simulink model "COMPLETETEST_InDividualLegControl"  (R2023a)
settings: Solver=VariableStepAuto  StartTime=0.0  StopTime=80.0  RelTol=1e-3
undefined symbols (not defined in the file or in its folder): X, Y, Z
libraries: sm_lib x95, simulink_extras x24, nesl_utility x10
(part 3 of 3)

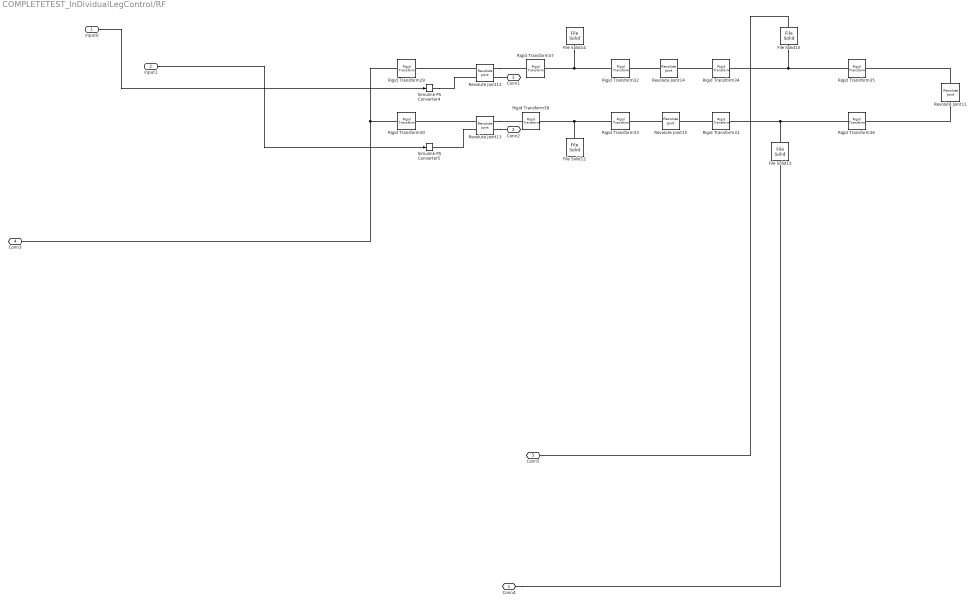
== system COMPLETETEST_InDividualLegControl/RF ==
  input0 : Inport
  input1 : Inport  Port=2
  File Solid12 : sm_lib/Body Elements/File Solid  ExtGeomFileName=F:\THE_LIBRARY\CODE_BASE\ROBOSERVO\Odrive\TINDALOS_THEDOG\SIM_MATLAB\ABSTARCT\LINK1.STL  UnitType=Custom  ExtGeomFileUnits=mm  StepReaderType=HEX  ExportConvexHullGeometry=off  InertiaType=CalculateFromGeometry  Mass=1  MassUnits=kg  CenterOfMass=[0 0 0]  CenterOfMassUnits=m  MomentsOfInertia=[1 1 1]  MomentsOfInertiaUnits=kg*m^2  ProductsOfInertia=[0 0 0]  ProductsOfInertiaUnits=kg*m^2  BasedOnType=Density  Density=1000  DensityUnits=kg/m^3  DoExposeReferenceFrame=on  SerializedFrames=<Frames/>  GraphicType=FromGeometry  MarkerShape=Sphere  MarkerSize=10  GraphicVisPropType=SimpleVisualProperties  GraphicDiffuseColor=[1.0 0.2 0.2]  GraphicSpecularColor=[0.5 0.5 0.5 1.0]  GraphicAmbientColor=[0.15 0.15 0.15 1.0]  GraphicEmissiveColor=[0.0 0.0 0.0 1.0]  GraphicShininess=75  GraphicOpacity=1.0
  File Solid13 : sm_lib/Body Elements/File Solid  ExtGeomFileName=F:\THE_LIBRARY\CODE_BASE\ROBOSERVO\Odrive\TINDALOS_THEDOG\SIM_MATLAB\ABSTARCT\LINK2.STL  UnitType=Custom  ExtGeomFileUnits=mm  StepReaderType=HEX  ExportConvexHullGeometry=on  InertiaType=CalculateFromGeometry  Mass=1  MassUnits=kg  CenterOfMass=[0 0 0]  CenterOfMassUnits=m  MomentsOfInertia=[1 1 1]  MomentsOfInertiaUnits=kg*m^2  ProductsOfInertia=[0 0 0]  ProductsOfInertiaUnits=kg*m^2  BasedOnType=Density  Density=1000  DensityUnits=kg/m^3  DoExposeReferenceFrame=on  SerializedFrames=<Frames/>  GraphicType=FromGeometry  MarkerShape=Sphere  MarkerSize=10  GraphicVisPropType=SimpleVisualProperties  GraphicDiffuseColor=[1.0 0.6 0.0]  GraphicSpecularColor=[0.5 0.5 0.5 1.0]  GraphicAmbientColor=[0.15 0.15 0.15 1.0]  GraphicEmissiveColor=[0.0 0.0 0.0 1.0]  GraphicShininess=75  GraphicOpacity=1.0
  File Solid14 : sm_lib/Body Elements/File Solid  ExtGeomFileName=F:\THE_LIBRARY\CODE_BASE\ROBOSERVO\Odrive\TINDALOS_THEDOG\SIM_MATLAB\ABSTARCT\LINK1.STL  UnitType=Custom  ExtGeomFileUnits=mm  StepReaderType=HEX  ExportConvexHullGeometry=off  InertiaType=CalculateFromGeometry  Mass=1  MassUnits=kg  CenterOfMass=[0 0 0]  CenterOfMassUnits=m  MomentsOfInertia=[1 1 1]  MomentsOfInertiaUnits=kg*m^2  ProductsOfInertia=[0 0 0]  ProductsOfInertiaUnits=kg*m^2  BasedOnType=Density  Density=1000  DensityUnits=kg/m^3  DoExposeReferenceFrame=on  SerializedFrames=<Frames/>  GraphicType=FromGeometry  MarkerShape=Sphere  MarkerSize=10  GraphicVisPropType=SimpleVisualProperties  GraphicDiffuseColor=[1.0 0.2 0.2]  GraphicSpecularColor=[0.5 0.5 0.5 1.0]  GraphicAmbientColor=[0.15 0.15 0.15 1.0]  GraphicEmissiveColor=[0.0 0.0 0.0 1.0]  GraphicShininess=75  GraphicOpacity=1.0
  File Solid15 : sm_lib/Body Elements/File Solid  ExtGeomFileName=F:\THE_LIBRARY\CODE_BASE\ROBOSERVO\Odrive\TINDALOS_THEDOG\SIM_MATLAB\ABSTARCT\LINK2.STL  UnitType=Custom  ExtGeomFileUnits=mm  StepReaderType=HEX  ExportConvexHullGeometry=on  InertiaType=CalculateFromGeometry  Mass=1  MassUnits=kg  CenterOfMass=[0 0 0]  CenterOfMassUnits=m  MomentsOfInertia=[1 1 1]  MomentsOfInertiaUnits=kg*m^2  ProductsOfInertia=[0 0 0]  ProductsOfInertiaUnits=kg*m^2  BasedOnType=Density  Density=1000  DensityUnits=kg/m^3  DoExposeReferenceFrame=on  SerializedFrames=<Frames/>  GraphicType=FromGeometry  MarkerShape=Sphere  MarkerSize=10  GraphicVisPropType=SimpleVisualProperties  GraphicDiffuseColor=[1.0 0.6 0.0]  GraphicSpecularColor=[0.5 0.5 0.5 1.0]  GraphicAmbientColor=[0.15 0.15 0.15 1.0]  GraphicEmissiveColor=[0.0 0.0 0.0 1.0]  GraphicShininess=75  GraphicOpacity=1.0
  Revolute Joint11 : sm_lib/Joints/Revolute Joint  JointMode=Normal  SenseConstraintForce=off  SenseConstraintForceX=off  SenseConstraintForceY=off  SenseConstraintForceZ=off  SenseConstraintTorque=off  SenseConstraintTorqueX=off  SenseConstraintTorqueY=off  SenseConstraintTorqueZ=off  SenseTotalForce=off  SenseTotalForceX=off  SenseTotalForceY=off  SenseTotalForceZ=off  SenseTotalTorque=off  SenseTotalTorqueX=off  SenseTotalTorqueY=off  SenseTotalTorqueZ=off  CompositeWrenchDir=FollowerOnBase  CompositeWrenchFrame=BaseFrame  EquilibriumPosition=0  EquilibriumPositionUnits=deg  SpringStiffness=0  SpringStiffnessUnits=N*m/deg  DampingCoefficient=0  DampingCoefficientUnits=N*m/(deg/s)  TorqueActuationMode=NoTorque  MotionActuationMode=ComputedMotion  SensePosition=off  SenseVelocity=off  SenseAcceleration=off  SenseTorqueForce=off  SenseLowerLimitTorqueForce=off  SenseUpperLimitTorqueForce=off  LowerLimitSpecify=off  LowerLimitBound=-90  LowerLimitBoundUnits=deg  LowerLimitStiffness=1e4  LowerLimitStiffnessUnits=N*m/deg  LowerLimitDamping=10  LowerLimitDampingUnits=N*m/(deg/s)  LowerLimitTransitionRegionWidth=0.1  LowerLimitTransitionRegionWidthUnits=deg  UpperLimitSpecify=off  UpperLimitBound=90  UpperLimitBoundUnits=deg  UpperLimitStiffness=1e4  UpperLimitStiffnessUnits=N*m/deg  UpperLimitDamping=10  UpperLimitDampingUnits=N*m/(deg/s)  UpperLimitTransitionRegionWidth=0.1  UpperLimitTransitionRegionWidthUnits=deg  PositionTargetSpecify=off  PositionTargetPriority=High  PositionTargetValue=0  PositionTargetValueUnits=deg  VelocityTargetSpecify=off  VelocityTargetPriority=High  VelocityTargetValue=0  VelocityTargetValueUnits=deg/s
  Revolute Joint12 : sm_lib/Joints/Revolute Joint  JointMode=Normal  SenseConstraintForce=off  SenseConstraintForceX=off  SenseConstraintForceY=off  SenseConstraintForceZ=off  SenseConstraintTorque=off  SenseConstraintTorqueX=off  SenseConstraintTorqueY=off  SenseConstraintTorqueZ=off  SenseTotalForce=off  SenseTotalForceX=off  SenseTotalForceY=off  SenseTotalForceZ=off  SenseTotalTorque=off  SenseTotalTorqueX=off  SenseTotalTorqueY=off  SenseTotalTorqueZ=off  CompositeWrenchDir=FollowerOnBase  CompositeWrenchFrame=BaseFrame  EquilibriumPosition=0  EquilibriumPositionUnits=deg  SpringStiffness=0  SpringStiffnessUnits=N*m/deg  DampingCoefficient=1e-4  DampingCoefficientUnits=N*m/(deg/s)  TorqueActuationMode=ComputedTorque  MotionActuationMode=InputMotion  SensePosition=on  SenseVelocity=off  SenseAcceleration=off  SenseTorqueForce=off  SenseLowerLimitTorqueForce=off  SenseUpperLimitTorqueForce=off  LowerLimitSpecify=off  LowerLimitBound=-90  LowerLimitBoundUnits=deg  LowerLimitStiffness=1e4  LowerLimitStiffnessUnits=N*m/deg  LowerLimitDamping=10  LowerLimitDampingUnits=N*m/(deg/s)  LowerLimitTransitionRegionWidth=0.1  LowerLimitTransitionRegionWidthUnits=deg  UpperLimitSpecify=off  UpperLimitBound=90  UpperLimitBoundUnits=deg  UpperLimitStiffness=1e4  UpperLimitStiffnessUnits=N*m/deg  UpperLimitDamping=10  UpperLimitDampingUnits=N*m/(deg/s)  UpperLimitTransitionRegionWidth=0.1  UpperLimitTransitionRegionWidthUnits=deg  PositionTargetSpecify=off  PositionTargetPriority=High  PositionTargetValue=120  PositionTargetValueUnits=deg  VelocityTargetSpecify=off  VelocityTargetPriority=High  VelocityTargetValue=0  VelocityTargetValueUnits=deg/s
  Revolute Joint13 : sm_lib/Joints/Revolute Joint  JointMode=Normal  SenseConstraintForce=off  SenseConstraintForceX=off  SenseConstraintForceY=off  SenseConstraintForceZ=off  SenseConstraintTorque=off  SenseConstraintTorqueX=off  SenseConstraintTorqueY=off  SenseConstraintTorqueZ=off  SenseTotalForce=off  SenseTotalForceX=off  SenseTotalForceY=off  SenseTotalForceZ=off  SenseTotalTorque=off  SenseTotalTorqueX=off  SenseTotalTorqueY=off  SenseTotalTorqueZ=off  CompositeWrenchDir=FollowerOnBase  CompositeWrenchFrame=BaseFrame  EquilibriumPosition=0  EquilibriumPositionUnits=deg  SpringStiffness=0  SpringStiffnessUnits=N*m/deg  DampingCoefficient=1e-4  DampingCoefficientUnits=N*m/(deg/s)  TorqueActuationMode=ComputedTorque  MotionActuationMode=InputMotion  SensePosition=on  SenseVelocity=off  SenseAcceleration=off  SenseTorqueForce=off  SenseLowerLimitTorqueForce=off  SenseUpperLimitTorqueForce=off  LowerLimitSpecify=off  LowerLimitBound=-90  LowerLimitBoundUnits=deg  LowerLimitStiffness=1e4  LowerLimitStiffnessUnits=N*m/deg  LowerLimitDamping=10  LowerLimitDampingUnits=N*m/(deg/s)  LowerLimitTransitionRegionWidth=0.1  LowerLimitTransitionRegionWidthUnits=deg  UpperLimitSpecify=off  UpperLimitBound=90  UpperLimitBoundUnits=deg  UpperLimitStiffness=1e4  UpperLimitStiffnessUnits=N*m/deg  UpperLimitDamping=10  UpperLimitDampingUnits=N*m/(deg/s)  UpperLimitTransitionRegionWidth=0.1  UpperLimitTransitionRegionWidthUnits=deg  PositionTargetSpecify=off  PositionTargetPriority=High  PositionTargetValue=-60  PositionTargetValueUnits=deg  VelocityTargetSpecify=off  VelocityTargetPriority=High  VelocityTargetValue=0  VelocityTargetValueUnits=deg/s
  Revolute Joint14 : sm_lib/Joints/Revolute Joint  JointMode=Normal  SenseConstraintForce=off  SenseConstraintForceX=off  SenseConstraintForceY=off  SenseConstraintForceZ=off  SenseConstraintTorque=off  SenseConstraintTorqueX=off  SenseConstraintTorqueY=off  SenseConstraintTorqueZ=off  SenseTotalForce=off  SenseTotalForceX=off  SenseTotalForceY=off  SenseTotalForceZ=off  SenseTotalTorque=off  SenseTotalTorqueX=off  SenseTotalTorqueY=off  SenseTotalTorqueZ=off  CompositeWrenchDir=FollowerOnBase  CompositeWrenchFrame=BaseFrame  EquilibriumPosition=0  EquilibriumPositionUnits=deg  SpringStiffness=0  SpringStiffnessUnits=N*m/deg  DampingCoefficient=0  DampingCoefficientUnits=N*m/(deg/s)  TorqueActuationMode=NoTorque  MotionActuationMode=ComputedMotion  SensePosition=off  SenseVelocity=off  SenseAcceleration=off  SenseTorqueForce=off  SenseLowerLimitTorqueForce=off  SenseUpperLimitTorqueForce=off  LowerLimitSpecify=off  LowerLimitBound=-90  LowerLimitBoundUnits=deg  LowerLimitStiffness=1e4  LowerLimitStiffnessUnits=N*m/deg  LowerLimitDamping=10  LowerLimitDampingUnits=N*m/(deg/s)  LowerLimitTransitionRegionWidth=0.1  LowerLimitTransitionRegionWidthUnits=deg  UpperLimitSpecify=off  UpperLimitBound=90  UpperLimitBoundUnits=deg  UpperLimitStiffness=1e4  UpperLimitStiffnessUnits=N*m/deg  UpperLimitDamping=10  UpperLimitDampingUnits=N*m/(deg/s)  UpperLimitTransitionRegionWidth=0.1  UpperLimitTransitionRegionWidthUnits=deg  PositionTargetSpecify=off  PositionTargetPriority=Low  PositionTargetValue=-135  PositionTargetValueUnits=deg  VelocityTargetSpecify=off  VelocityTargetPriority=High  VelocityTargetValue=90  VelocityTargetValueUnits=deg/s
  Revolute Joint15 : sm_lib/Joints/Revolute Joint  JointMode=Normal  SenseConstraintForce=off  SenseConstraintForceX=off  SenseConstraintForceY=off  SenseConstraintForceZ=off  SenseConstraintTorque=off  SenseConstraintTorqueX=off  SenseConstraintTorqueY=off  SenseConstraintTorqueZ=off  SenseTotalForce=off  SenseTotalForceX=off  SenseTotalForceY=off  SenseTotalForceZ=off  SenseTotalTorque=off  SenseTotalTorqueX=off  SenseTotalTorqueY=off  SenseTotalTorqueZ=off  CompositeWrenchDir=FollowerOnBase  CompositeWrenchFrame=BaseFrame  EquilibriumPosition=0  EquilibriumPositionUnits=deg  SpringStiffness=0  SpringStiffnessUnits=N*m/deg  DampingCoefficient=0  DampingCoefficientUnits=N*m/(deg/s)  TorqueActuationMode=NoTorque  MotionActuationMode=ComputedMotion  SensePosition=off  SenseVelocity=off  SenseAcceleration=off  SenseTorqueForce=off  SenseLowerLimitTorqueForce=off  SenseUpperLimitTorqueForce=off  LowerLimitSpecify=off  LowerLimitBound=-90  LowerLimitBoundUnits=deg  LowerLimitStiffness=1e4  LowerLimitStiffnessUnits=N*m/deg  LowerLimitDamping=10  LowerLimitDampingUnits=N*m/(deg/s)  LowerLimitTransitionRegionWidth=0.1  LowerLimitTransitionRegionWidthUnits=deg  UpperLimitSpecify=off  UpperLimitBound=90  UpperLimitBoundUnits=deg  UpperLimitStiffness=1e4  UpperLimitStiffnessUnits=N*m/deg  UpperLimitDamping=10  UpperLimitDampingUnits=N*m/(deg/s)  UpperLimitTransitionRegionWidth=0.1  UpperLimitTransitionRegionWidthUnits=deg  PositionTargetSpecify=off  PositionTargetPriority=Low  PositionTargetValue=-135  PositionTargetValueUnits=deg  VelocityTargetSpecify=off  VelocityTargetPriority=High  VelocityTargetValue=90  VelocityTargetValueUnits=deg/s
  Rigid Transform29 : sm_lib/Frames and Transforms/Rigid Transform  TranslationMethod=StandardAxis  TranslationStandardOffset=6  TranslationStandardOffsetUnits=mm  TranslationStandardAxis=+Z  TranslationCartesianOffset=[0 0 0]  TranslationCartesianOffsetUnits=m  TranslationROffset=0  TranslationROffsetUnits=m  TranslationZOffset=0  TranslationZOffsetUnits=m  TranslationThetaOffset=0  TranslationThetaOffsetUnits=deg  RotationMethod=None  RotationAngleUnits=deg  RotationStandardAxis=+X  RotationAngle=90  RotationArbitraryAxis=[0 0 1]  FollAlignAxisA=+X  BaseAlignAxisA=+Y  FollAlignAxisB=+Y  BaseAlignAxisB=+Z  RotationSequenceAxes=FollowerAxes  RotationSequence=XYX  RotationSequenceAngles=[0 0 0]  RotationSequenceAnglesUnits=deg  RotationMatrix=[1 0 0; 0 1 0; 0 0 1]  Quaternion=[1 0 0 0]
  Rigid Transform30 : sm_lib/Frames and Transforms/Rigid Transform  TranslationMethod=StandardAxis  TranslationStandardOffset=6  TranslationStandardOffsetUnits=mm  TranslationStandardAxis=-Z  TranslationCartesianOffset=[0 0 0]  TranslationCartesianOffsetUnits=m  TranslationROffset=0  TranslationROffsetUnits=m  TranslationZOffset=0  TranslationZOffsetUnits=m  TranslationThetaOffset=0  TranslationThetaOffsetUnits=deg  RotationMethod=None  RotationAngleUnits=deg  RotationStandardAxis=+X  RotationAngle=90  RotationArbitraryAxis=[0 0 1]  FollAlignAxisA=+X  BaseAlignAxisA=+Y  FollAlignAxisB=+Y  BaseAlignAxisB=+Z  RotationSequenceAxes=FollowerAxes  RotationSequence=XYX  RotationSequenceAngles=[0 0 0]  RotationSequenceAnglesUnits=deg  RotationMatrix=[1 0 0; 0 1 0; 0 0 1]  Quaternion=[1 0 0 0]
  Rigid Transform31 : sm_lib/Frames and Transforms/Rigid Transform  TranslationMethod=StandardAxis  TranslationStandardOffset=6  TranslationStandardOffsetUnits=mm  TranslationStandardAxis=-Z  TranslationCartesianOffset=[0 0 0]  TranslationCartesianOffsetUnits=m  TranslationROffset=0  TranslationROffsetUnits=m  TranslationZOffset=0  TranslationZOffsetUnits=m  TranslationThetaOffset=0  TranslationThetaOffsetUnits=deg  RotationMethod=StandardAxis  RotationAngleUnits=deg  RotationStandardAxis=+X  RotationAngle=-90  RotationArbitraryAxis=[0 0 1]  FollAlignAxisA=+X  BaseAlignAxisA=+Y  FollAlignAxisB=+Y  BaseAlignAxisB=+Z  RotationSequenceAxes=FollowerAxes  RotationSequence=XYX  RotationSequenceAngles=[0 0 0]  RotationSequenceAnglesUnits=deg  RotationMatrix=[1 0 0; 0 1 0; 0 0 1]  Quaternion=[1 0 0 0]
  Rigid Transform32 : sm_lib/Frames and Transforms/Rigid Transform  TranslationMethod=StandardAxis  TranslationStandardOffset=100  TranslationStandardOffsetUnits=mm  TranslationStandardAxis=-Z  TranslationCartesianOffset=[0 0 0]  TranslationCartesianOffsetUnits=mm  TranslationROffset=0  TranslationROffsetUnits=m  TranslationZOffset=0  TranslationZOffsetUnits=m  TranslationThetaOffset=0  TranslationThetaOffsetUnits=deg  RotationMethod=StandardAxis  RotationAngleUnits=deg  RotationStandardAxis=+X  RotationAngle=90  RotationArbitraryAxis=[0 0 1]  FollAlignAxisA=+X  BaseAlignAxisA=+Y  FollAlignAxisB=+Y  BaseAlignAxisB=+Z  RotationSequenceAxes=FollowerAxes  RotationSequence=XYX  RotationSequenceAngles=[0 0 0]  RotationSequenceAnglesUnits=deg  RotationMatrix=[1 0 0; 0 1 0; 0 0 1]  Quaternion=[1 0 0 0]
  Rigid Transform33 : sm_lib/Frames and Transforms/Rigid Transform  TranslationMethod=StandardAxis  TranslationStandardOffset=100  TranslationStandardOffsetUnits=mm  TranslationStandardAxis=-Z  TranslationCartesianOffset=[0 0 0]  TranslationCartesianOffsetUnits=mm  TranslationROffset=0  TranslationROffsetUnits=m  TranslationZOffset=0  TranslationZOffsetUnits=m  TranslationThetaOffset=0  TranslationThetaOffsetUnits=deg  RotationMethod=StandardAxis  RotationAngleUnits=deg  RotationStandardAxis=+X  RotationAngle=90  RotationArbitraryAxis=[0 0 1]  FollAlignAxisA=+X  BaseAlignAxisA=+Y  FollAlignAxisB=+Y  BaseAlignAxisB=+Z  RotationSequenceAxes=FollowerAxes  RotationSequence=XYX  RotationSequenceAngles=[0 0 0]  RotationSequenceAnglesUnits=deg  RotationMatrix=[1 0 0; 0 1 0; 0 0 1]  Quaternion=[1 0 0 0]
  Rigid Transform34 : sm_lib/Frames and Transforms/Rigid Transform  TranslationMethod=StandardAxis  TranslationStandardOffset=6  TranslationStandardOffsetUnits=mm  TranslationStandardAxis=+Z  TranslationCartesianOffset=[0 0 0]  TranslationCartesianOffsetUnits=m  TranslationROffset=0  TranslationROffsetUnits=m  TranslationZOffset=0  TranslationZOffsetUnits=m  TranslationThetaOffset=0  TranslationThetaOffsetUnits=deg  RotationMethod=StandardAxis  RotationAngleUnits=deg  RotationStandardAxis=+X  RotationAngle=-90  RotationArbitraryAxis=[0 0 1]  FollAlignAxisA=+X  BaseAlignAxisA=+Y  FollAlignAxisB=+Y  BaseAlignAxisB=+Z  RotationSequenceAxes=FollowerAxes  RotationSequence=XYX  RotationSequenceAngles=[0 0 0]  RotationSequenceAnglesUnits=deg  RotationMatrix=[1 0 0; 0 1 0; 0 0 1]  Quaternion=[1 0 0 0]
  Rigid Transform35 : sm_lib/Frames and Transforms/Rigid Transform  TranslationMethod=Cartesian  TranslationStandardOffset=180  TranslationStandardOffsetUnits=mm  TranslationStandardAxis=-Z  TranslationCartesianOffset=[0 12 -180]  TranslationCartesianOffsetUnits=mm  TranslationROffset=0  TranslationROffsetUnits=m  TranslationZOffset=0  TranslationZOffsetUnits=m  TranslationThetaOffset=0  TranslationThetaOffsetUnits=deg  RotationMethod=StandardAxis  RotationAngleUnits=deg  RotationStandardAxis=+X  RotationAngle=90  RotationArbitraryAxis=[0 0 1]  FollAlignAxisA=+X  BaseAlignAxisA=+Y  FollAlignAxisB=+Y  BaseAlignAxisB=+Z  RotationSequenceAxes=FollowerAxes  RotationSequence=XYX  RotationSequenceAngles=[0 0 0]  RotationSequenceAnglesUnits=deg  RotationMatrix=[1 0 0; 0 1 0; 0 0 1]  Quaternion=[1 0 0 0]
  Rigid Transform36 : sm_lib/Frames and Transforms/Rigid Transform  TranslationMethod=Cartesian  TranslationStandardOffset=180  TranslationStandardOffsetUnits=mm  TranslationStandardAxis=-Z  TranslationCartesianOffset=[0 -12 -180]  TranslationCartesianOffsetUnits=mm  TranslationROffset=0  TranslationROffsetUnits=m  TranslationZOffset=0  TranslationZOffsetUnits=m  TranslationThetaOffset=0  TranslationThetaOffsetUnits=deg  RotationMethod=StandardAxis  RotationAngleUnits=deg  RotationStandardAxis=+X  RotationAngle=90  RotationArbitraryAxis=[0 0 1]  FollAlignAxisA=+X  BaseAlignAxisA=+Y  FollAlignAxisB=+Y  BaseAlignAxisB=+Z  RotationSequenceAxes=FollowerAxes  RotationSequence=XYX  RotationSequenceAngles=[0 0 0]  RotationSequenceAnglesUnits=deg  RotationMatrix=[1 0 0; 0 1 0; 0 0 1]  Quaternion=[1 0 0 0]
  Rigid Transform37 : sm_lib/Frames and Transforms/Rigid Transform  TranslationMethod=None  TranslationStandardOffset=6  TranslationStandardOffsetUnits=mm  TranslationStandardAxis=+Y  TranslationCartesianOffset=[0 0 0]  TranslationCartesianOffsetUnits=m  TranslationROffset=0  TranslationROffsetUnits=m  TranslationZOffset=0  TranslationZOffsetUnits=m  TranslationThetaOffset=0  TranslationThetaOffsetUnits=deg  RotationMethod=StandardAxis  RotationAngleUnits=deg  RotationStandardAxis=+X  RotationAngle=-90  RotationArbitraryAxis=[0 0 1]  FollAlignAxisA=+X  BaseAlignAxisA=+Y  FollAlignAxisB=+Y  BaseAlignAxisB=+Z  RotationSequenceAxes=FollowerAxes  RotationSequence=XYX  RotationSequenceAngles=[0 0 0]  RotationSequenceAnglesUnits=deg  RotationMatrix=[1 0 0; 0 1 0; 0 0 1]  Quaternion=[1 0 0 0]
  Rigid Transform38 : sm_lib/Frames and Transforms/Rigid Transform  TranslationMethod=None  TranslationStandardOffset=6  TranslationStandardOffsetUnits=mm  TranslationStandardAxis=+Y  TranslationCartesianOffset=[0 0 0]  TranslationCartesianOffsetUnits=m  TranslationROffset=0  TranslationROffsetUnits=m  TranslationZOffset=0  TranslationZOffsetUnits=m  TranslationThetaOffset=0  TranslationThetaOffsetUnits=deg  RotationMethod=StandardAxis  RotationAngleUnits=deg  RotationStandardAxis=+X  RotationAngle=-90  RotationArbitraryAxis=[0 0 1]  FollAlignAxisA=+X  BaseAlignAxisA=+Y  FollAlignAxisB=+Y  BaseAlignAxisB=+Z  RotationSequenceAxes=FollowerAxes  RotationSequence=XYX  RotationSequenceAngles=[0 0 0]  RotationSequenceAnglesUnits=deg  RotationMatrix=[1 0 0; 0 1 0; 0 0 1]  Quaternion=[1 0 0 0]
  Simulink-PS Converter4 : nesl_utility/Simulink-PS Converter  PhysicalDomain=network_engine_domain  SubClassName=ps_input  LeftPortType=input  RightPortType=output  PseudoPeriodic=off  Frequencies=[]  NoiseDistribution=none  NoiseParameters=[]  Unit=1  AffineConversion=off  FilteringAndDerivatives=filter  SimscapeFilterOrder=2  InputFilterTimeConstant=0.001  UdotUserProvided=0
  Simulink-PS Converter5 : nesl_utility/Simulink-PS Converter  PhysicalDomain=network_engine_domain  SubClassName=ps_input  LeftPortType=input  RightPortType=output  PseudoPeriodic=off  Frequencies=[]  NoiseDistribution=none  NoiseParameters=[]  Unit=1  AffineConversion=off  FilteringAndDerivatives=filter  SimscapeFilterOrder=2  InputFilterTimeConstant=0.001  UdotUserProvided=0
  Conn4 : PMIOPort  Side=Left
  Conn2 : PMIOPort  Port=2  Side=Right
  Conn1 : PMIOPort  Port=3  Side=Right
  Conn3 : PMIOPort  Port=4  Side=Right
  Conn5 : PMIOPort  Port=5  Side=Left
  wires:
  input1/1 -> Simulink-PS Converter5/1
  input0/1 -> Simulink-PS Converter4/1
  connections:
  File Solid12/RConn1 -- Rigid Transform33/LConn1 -- Rigid Transform38/RConn1
  Rigid Transform31/LConn1 -- Revolute Joint15/RConn1
  Simulink-PS Converter4/RConn1 -- Revolute Joint12/LConn2
  Revolute Joint13/LConn2 -- Simulink-PS Converter5/RConn1
  Revolute Joint11/RConn1 -- Rigid Transform35/RConn1
  Rigid Transform31/RConn1 -- Rigid Transform36/LConn1 -- File Solid13/RConn1
  Rigid Transform35/LConn1 -- Rigid Transform34/RConn1 -- File Solid15/RConn1
  Revolute Joint13/LConn1 -- Rigid Transform30/RConn1
  Revolute Joint14/LConn1 -- Rigid Transform32/RConn1
  File Solid14/RConn1 -- Rigid Transform32/LConn1 -- Rigid Transform37/RConn1
  Rigid Transform29/RConn1 -- Revolute Joint12/LConn1
  Revolute Joint12/RConn2 -- Conn1/RConn1
  Rigid Transform29/LConn1 -- Rigid Transform30/LConn1 -- Conn3/RConn1
  Revolute Joint12/RConn1 -- Rigid Transform37/LConn1
  Revolute Joint11/LConn1 -- Rigid Transform36/RConn1
  Rigid Transform34/LConn1 -- Revolute Joint14/RConn1
  Revolute Joint13/RConn1 -- Rigid Transform38/LConn1
  Revolute Joint15/LConn1 -- Rigid Transform33/RConn1
  Conn4/RConn1 -- File Solid13/LConn1
  Revolute Joint13/RConn2 -- Conn2/RConn1
  File Solid15/LConn1 -- Conn5/RConn1

== system COMPLETETEST_InDividualLegControl/Subsystem3 ==
  Subsystem : Subsystem
  Subsystem7 : Subsystem
  u : Outport
  u1 : Outport  Port=2
  wires:
  Subsystem7/1(u) -> u/1
  Subsystem/1(u) -> u1/1

== system COMPLETETEST_InDividualLegControl/Subsystem4 ==
  Subsystem : Subsystem
  Subsystem7 : Subsystem
  u : Outport
  u1 : Outport  Port=2
  wires:
  Subsystem7/1(u) -> u/1
  Subsystem/1(u) -> u1/1

== system COMPLETETEST_InDividualLegControl/Subsystem7 ==
  Subsystem : Subsystem
  Subsystem7 : Subsystem
  u : Outport
  u1 : Outport  Port=2
  wires:
  Subsystem7/1(u) -> u/1
  Subsystem/1(u) -> u1/1

== system COMPLETETEST_InDividualLegControl/Subsystem8 ==
  Subsystem : Subsystem
  Subsystem7 : Subsystem
  u : Outport
  u1 : Outport  Port=2
  wires:
  Subsystem7/1(u) -> u/1
  Subsystem/1(u) -> u1/1

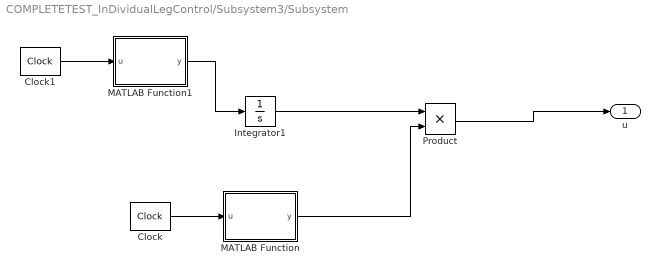
== system COMPLETETEST_InDividualLegControl/Subsystem3/Subsystem ==
  Clock : simulink_extras/Flip Flops/Clock  period=4
  Clock1 : simulink_extras/Flip Flops/Clock  period=2
  Integrator1 : Integrator
  MATLAB Function : MATLAB Function  TreatAsAtomicUnit=on
  MATLAB Function1 : MATLAB Function  TreatAsAtomicUnit=on
  Product : Product
  u : Outport  VectorParamsAs1DForOutWhenUnconnected=off
  wires:
  MATLAB Function1/1(y) -> Integrator1/1
  Clock1/1 -> MATLAB Function1/1(u)
  MATLAB Function/1(y) -> Product/2
  Clock/1 -> MATLAB Function/1(u)
  Integrator1/1 -> Product/1
  Product/1 -> u/1

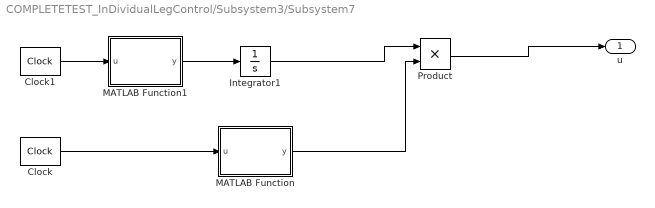
== system COMPLETETEST_InDividualLegControl/Subsystem3/Subsystem7 ==
  Clock : simulink_extras/Flip Flops/Clock  period=8
  Clock1 : simulink_extras/Flip Flops/Clock  period=4
  Integrator1 : Integrator
  MATLAB Function : MATLAB Function  TreatAsAtomicUnit=on
  MATLAB Function1 : MATLAB Function  TreatAsAtomicUnit=on
  Product : Product
  u : Outport  VectorParamsAs1DForOutWhenUnconnected=off
  wires:
  MATLAB Function1/1(y) -> Integrator1/1
  Clock1/1 -> MATLAB Function1/1(u)
  MATLAB Function/1(y) -> Product/2
  Clock/1 -> MATLAB Function/1(u)
  Integrator1/1 -> Product/1
  Product/1 -> u/1

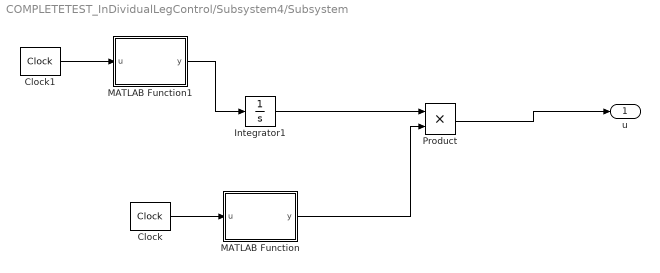
== system COMPLETETEST_InDividualLegControl/Subsystem4/Subsystem ==
  Clock : simulink_extras/Flip Flops/Clock  period=4
  Clock1 : simulink_extras/Flip Flops/Clock  period=2
  Integrator1 : Integrator
  MATLAB Function : MATLAB Function  TreatAsAtomicUnit=on
  MATLAB Function1 : MATLAB Function  TreatAsAtomicUnit=on
  Product : Product
  u : Outport  VectorParamsAs1DForOutWhenUnconnected=off
  wires:
  MATLAB Function1/1(y) -> Integrator1/1
  Clock1/1 -> MATLAB Function1/1(u)
  MATLAB Function/1(y) -> Product/2
  Clock/1 -> MATLAB Function/1(u)
  Integrator1/1 -> Product/1
  Product/1 -> u/1

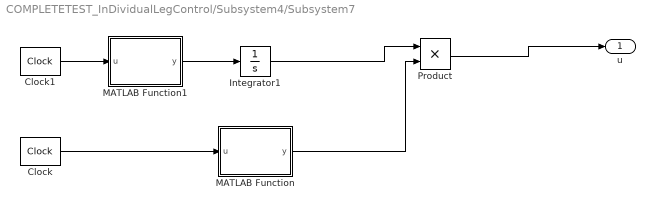
== system COMPLETETEST_InDividualLegControl/Subsystem4/Subsystem7 ==
  Clock : simulink_extras/Flip Flops/Clock  period=8
  Clock1 : simulink_extras/Flip Flops/Clock  period=4
  Integrator1 : Integrator
  MATLAB Function : MATLAB Function  TreatAsAtomicUnit=on
  MATLAB Function1 : MATLAB Function  TreatAsAtomicUnit=on
  Product : Product
  u : Outport  VectorParamsAs1DForOutWhenUnconnected=off
  wires:
  MATLAB Function1/1(y) -> Integrator1/1
  Clock1/1 -> MATLAB Function1/1(u)
  MATLAB Function/1(y) -> Product/2
  Clock/1 -> MATLAB Function/1(u)
  Integrator1/1 -> Product/1
  Product/1 -> u/1

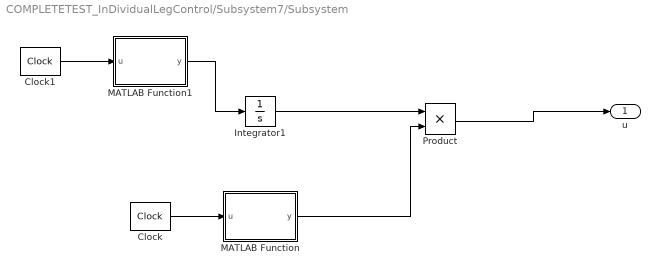
== system COMPLETETEST_InDividualLegControl/Subsystem7/Subsystem ==
  Clock : simulink_extras/Flip Flops/Clock  period=4
  Clock1 : simulink_extras/Flip Flops/Clock  period=2
  Integrator1 : Integrator
  MATLAB Function : MATLAB Function  TreatAsAtomicUnit=on
  MATLAB Function1 : MATLAB Function  TreatAsAtomicUnit=on
  Product : Product
  u : Outport  VectorParamsAs1DForOutWhenUnconnected=off
  wires:
  MATLAB Function1/1(y) -> Integrator1/1
  Clock1/1 -> MATLAB Function1/1(u)
  MATLAB Function/1(y) -> Product/2
  Clock/1 -> MATLAB Function/1(u)
  Integrator1/1 -> Product/1
  Product/1 -> u/1

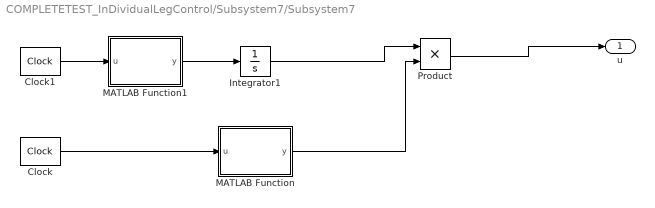
== system COMPLETETEST_InDividualLegControl/Subsystem7/Subsystem7 ==
  Clock : simulink_extras/Flip Flops/Clock  period=8
  Clock1 : simulink_extras/Flip Flops/Clock  period=4
  Integrator1 : Integrator
  MATLAB Function : MATLAB Function  TreatAsAtomicUnit=on
  MATLAB Function1 : MATLAB Function  TreatAsAtomicUnit=on
  Product : Product
  u : Outport  VectorParamsAs1DForOutWhenUnconnected=off
  wires:
  MATLAB Function1/1(y) -> Integrator1/1
  Clock1/1 -> MATLAB Function1/1(u)
  MATLAB Function/1(y) -> Product/2
  Clock/1 -> MATLAB Function/1(u)
  Integrator1/1 -> Product/1
  Product/1 -> u/1

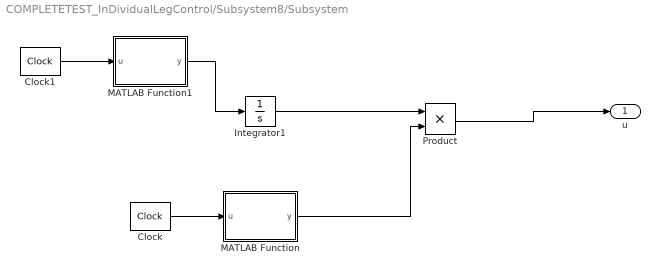
== system COMPLETETEST_InDividualLegControl/Subsystem8/Subsystem ==
  Clock : simulink_extras/Flip Flops/Clock  period=4
  Clock1 : simulink_extras/Flip Flops/Clock  period=2
  Integrator1 : Integrator
  MATLAB Function : MATLAB Function  TreatAsAtomicUnit=on
  MATLAB Function1 : MATLAB Function  TreatAsAtomicUnit=on
  Product : Product
  u : Outport  VectorParamsAs1DForOutWhenUnconnected=off
  wires:
  MATLAB Function1/1(y) -> Integrator1/1
  Clock1/1 -> MATLAB Function1/1(u)
  MATLAB Function/1(y) -> Product/2
  Clock/1 -> MATLAB Function/1(u)
  Integrator1/1 -> Product/1
  Product/1 -> u/1

== system COMPLETETEST_InDividualLegControl/Subsystem8/Subsystem7 ==
  Clock : simulink_extras/Flip Flops/Clock  period=8
  Clock1 : simulink_extras/Flip Flops/Clock  period=4
  Integrator1 : Integrator
  MATLAB Function : MATLAB Function  TreatAsAtomicUnit=on
  MATLAB Function1 : MATLAB Function  TreatAsAtomicUnit=on
  Product : Product
  u : Outport  VectorParamsAs1DForOutWhenUnconnected=off
  wires:
  MATLAB Function1/1(y) -> Integrator1/1
  Clock1/1 -> MATLAB Function1/1(u)
  MATLAB Function/1(y) -> Product/2
  Clock/1 -> MATLAB Function/1(u)
  Integrator1/1 -> Product/1
  Product/1 -> u/1

== matlab function COMPLETETEST_InDividualLegControl/0-Tm_y3 ==
  data: u input; y output; S input; Tm input; H input
function y = fcn(u,S,Tm,H)

n=4;
if u>0
    y=2*H*(u/Tm-1/(n*pi)*sin(n*pi*u/Tm)).*(u>=0&u<Tm/2)+2*H*(1-u/Tm+1/(n*pi)*sin(n*pi*u/Tm)).*(u>=Tm/2&u<Tm);;
else 
    y=0;
end

== matlab function COMPLETETEST_InDividualLegControl/0-Tm_x1 ==
  data: u input; x output; Tm input; S input
function x = fcn(u,Tm,S)

if u>0
    x =S*(u/Tm-1/(2*pi)*sin(2*pi*u/Tm));
else 
    u=-u;
     x =S*(u/Tm-1/(2*pi)*sin(2*pi*u/Tm));
end

== matlab function COMPLETETEST_InDividualLegControl/0-Tm_x5 ==
  data: u input; x output; t input; y output
function [x,y]  = fcn(u,t)

if u>0
    x= u;
    y= t;
else 
    x = -u;
    y = 0;
end

== matlab function COMPLETETEST_InDividualLegControl/0-Tm_x4 ==
  data: u input; x output; Tm input; S input
function x = fcn(u,Tm,S)

if u>0
    x =S*(u/Tm-1/(2*pi)*sin(2*pi*u/Tm));
else 
    u=-u;
     x =S*(u/Tm-1/(2*pi)*sin(2*pi*u/Tm));
end

== matlab function COMPLETETEST_InDividualLegControl/0-Tm_y4 ==
  data: u input; y output; S input; Tm input; H input
function y = fcn(u,S,Tm,H)

n=4;
if u>0
    y=2*H*(u/Tm-1/(n*pi)*sin(n*pi*u/Tm)).*(u>=0&u<Tm/2)+2*H*(1-u/Tm+1/(n*pi)*sin(n*pi*u/Tm)).*(u>=Tm/2&u<Tm);;
else 
    y=0;
end

== matlab function COMPLETETEST_InDividualLegControl/Subsystem4/Subsystem7/MATLAB Function ==
  data: u input; y output
function y = fcn(u)
if u==0
    y = -1;
else
    y=1;
end
end

== matlab function COMPLETETEST_InDividualLegControl/Subsystem4/Subsystem7/MATLAB Function1 ==
  data: u input; y output
function y = fcn(u)
if u==0
    y = -1;
else
    y=1;
end
end

== matlab function COMPLETETEST_InDividualLegControl/Subsystem3/Subsystem/MATLAB Function ==
  data: u input; y output
function y = fcn(u)
if u==0
    y = -1;
else
    y=1;
end
end

== matlab function COMPLETETEST_InDividualLegControl/Subsystem3/Subsystem/MATLAB Function1 ==
  data: u input; y output
function y = fcn(u)
if u==0
    y = -1;
else
    y=1;
end
end

== matlab function COMPLETETEST_InDividualLegControl/Subsystem3/Subsystem7/MATLAB Function ==
  data: u input; y output
function y = fcn(u)
if u==0
    y = -1;
else
    y=1;
end
end

== matlab function COMPLETETEST_InDividualLegControl/Subsystem3/Subsystem7/MATLAB Function1 ==
  data: u input; y output
function y = fcn(u)
if u==0
    y = -1;
else
    y=1;
end
end

== matlab function COMPLETETEST_InDividualLegControl/Subsystem7/Subsystem/MATLAB Function ==
  data: u input; y output
function y = fcn(u)
if u==0
    y = -1;
else
    y=1;
end
end

== matlab function COMPLETETEST_InDividualLegControl/Subsystem7/Subsystem/MATLAB Function1 ==
  data: u input; y output
function y = fcn(u)
if u==0
    y = -1;
else
    y=1;
end
end

== matlab function COMPLETETEST_InDividualLegControl/0-Tm_y2 ==
  data: u input; y output; S input; Tm input; H input
function y = fcn(u,S,Tm,H)

n=4;
if u>0
    y=2*H*(u/Tm-1/(n*pi)*sin(n*pi*u/Tm)).*(u>=0&u<Tm/2)+2*H*(1-u/Tm+1/(n*pi)*sin(n*pi*u/Tm)).*(u>=Tm/2&u<Tm);;
else 
    y=0;
end

== matlab function COMPLETETEST_InDividualLegControl/Subsystem7/Subsystem7/MATLAB Function ==
  data: u input; y output
function y = fcn(u)
if u==0
    y = -1;
else
    y=1;
end
end

== matlab function COMPLETETEST_InDividualLegControl/Subsystem7/Subsystem7/MATLAB Function1 ==
  data: u input; y output
function y = fcn(u)
if u==0
    y = -1;
else
    y=1;
end
end

== matlab function COMPLETETEST_InDividualLegControl/Subsystem8/Subsystem/MATLAB Function ==
  data: u input; y output
function y = fcn(u)
if u==0
    y = -1;
else
    y=1;
end
end

== matlab function COMPLETETEST_InDividualLegControl/Subsystem8/Subsystem/MATLAB Function1 ==
  data: u input; y output
function y = fcn(u)
if u==0
    y = -1;
else
    y=1;
end
end

== matlab function COMPLETETEST_InDividualLegControl/Subsystem8/Subsystem7/MATLAB Function ==
  data: u input; y output
function y = fcn(u)
if u==0
    y = -1;
else
    y=1;
end
end

== matlab function COMPLETETEST_InDividualLegControl/Subsystem8/Subsystem7/MATLAB Function1 ==
  data: u input; y output
function y = fcn(u)
if u==0
    y = -1;
else
    y=1;
end
end

== matlab function COMPLETETEST_InDividualLegControl/MATLAB Function ==
  data: x1 input; theta_OUT output; z1 input; theta_IN output
function [theta_OUT, theta_IN ] = fcn(x1, z1)

%#codegen


L1 = 100;
L2 = 180;

x = x1;
y = z1;

L = sqrt(x^2 + y^2);

theta_left =  rad2deg(asin(x/L));

theta_right = rad2deg( acos((L^2 + L1^2-L2^2)/(2*L1*L)));



theta_OUT = theta_right- theta_left ;

theta_IN = theta_right + theta_left;

== matlab function COMPLETETEST_InDividualLegControl/0-Tm_x2 ==
  data: u input; x output; Tm input; S input
function x = fcn(u,Tm,S)

if u>0
    x =S*(u/Tm-1/(2*pi)*sin(2*pi*u/Tm));
else 
    u=-u;
     x =S*(u/Tm-1/(2*pi)*sin(2*pi*u/Tm));
end

== matlab function COMPLETETEST_InDividualLegControl/0-Tm_y1 ==
  data: u input; y output; S input; Tm input; H input
function y = fcn(u,S,Tm,H)

n=4;
if u>0
    y=2*H*(u/Tm-1/(n*pi)*sin(n*pi*u/Tm)).*(u>=0&u<Tm/2)+2*H*(1-u/Tm+1/(n*pi)*sin(n*pi*u/Tm)).*(u>=Tm/2&u<Tm);;
else 
    y=0;
end

== matlab function COMPLETETEST_InDividualLegControl/MATLAB Function1 ==
  data: x1 input; theta_OUT output; z1 input; theta_IN output
function [theta_OUT, theta_IN ] = fcn(x1, z1)

%#codegen


L1 = 100;
L2 = 180;

x = x1;
y = z1;

L = sqrt(x^2 + y^2);

theta_left =  rad2deg(asin(x/L));

theta_right = rad2deg( acos((L^2 + L1^2-L2^2)/(2*L1*L)));



theta_OUT = theta_right- theta_left ;

theta_IN = theta_right + theta_left;

== matlab function COMPLETETEST_InDividualLegControl/MATLAB Function2 ==
  data: x1 input; theta_OUT output; z1 input; theta_IN output
function [theta_OUT, theta_IN ] = fcn(x1, z1)

%#codegen


L1 = 100;
L2 = 180;

x = x1;
y = z1;

L = sqrt(x^2 + y^2);

theta_left =  rad2deg(asin(x/L));

theta_right = rad2deg( acos((L^2 + L1^2-L2^2)/(2*L1*L)));



theta_OUT = theta_right- theta_left ;

theta_IN = theta_right + theta_left;

== matlab function COMPLETETEST_InDividualLegControl/MATLAB Function3 ==
  data: x1 input; theta_OUT output; z1 input; theta_IN output
function [theta_OUT, theta_IN ] = fcn(x1, z1)

%#codegen


L1 = 100;
L2 = 180;

x = x1;
y = z1;

L = sqrt(x^2 + y^2);

theta_left =  rad2deg(asin(x/L));

theta_right = rad2deg( acos((L^2 + L1^2-L2^2)/(2*L1*L)));



theta_OUT = theta_right- theta_left ;

theta_IN = theta_right + theta_left;

== matlab function COMPLETETEST_InDividualLegControl/Subsystem4/Subsystem/MATLAB Function ==
  data: u input; y output
function y = fcn(u)
if u==0
    y = -1;
else
    y=1;
end
end

== matlab function COMPLETETEST_InDividualLegControl/Subsystem4/Subsystem/MATLAB Function1 ==
  data: u input; y output
function y = fcn(u)
if u==0
    y = -1;
else
    y=1;
end
end

== matlab function COMPLETETEST_InDividualLegControl/0-Tm_x3 ==
  data: u input; x output; Tm input; S input
function x = fcn(u,Tm,S)

if u>0
    x =S*(u/Tm-1/(2*pi)*sin(2*pi*u/Tm));
else 
    u=-u;
     x =S*(u/Tm-1/(2*pi)*sin(2*pi*u/Tm));
end
